simulink model "washing"  (R2024b)
settings: Solver=VariableStepAuto  StartTime=0.0  StopTime=inf  RelTol=1e-3
settings Model: Creator=Dell  LastModifiedBy=Dell

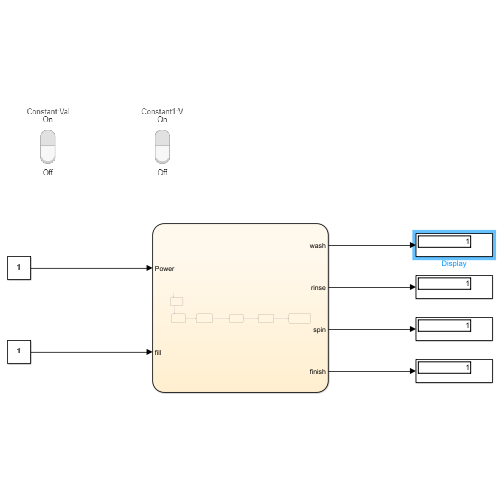
[thumbnail: Simulink's stored preview of the top-level diagram]
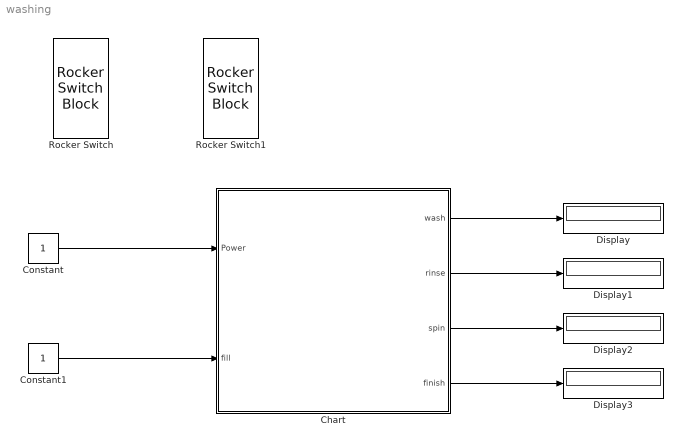
== system washing ==
  Chart : Stateflow chart  TreatAsAtomicUnit=on
  Constant : Constant
  Constant1 : Constant
  Display{,1..3} (4 alike) : Display
  Rocker Switch : RockerSwitchBlock
      settings: Values={{'Off', 'On'}, [0 1]}
  Rocker Switch1 : RockerSwitchBlock
      settings: Values={{'Off', 'On'}, [0 1]}
  wires:
  Constant/1 -> Chart/1(Power)
  Constant1/1 -> Chart/2(fill)
  Chart/2(rinse) -> Display1/1
  Chart/3(spin) -> Display2/1
  Chart/4(finish) -> Display3/1
  Chart/1(wash) -> Display/1

== stateflow chart washing/Chart ==
  state Power_on
  state finish
    entry:finish=1
  state wash
    entry:wash=1
  state fill
  state rinse
    entry:rinse=1
  state spin
    entry:spin=1
  (default) -> Power_on
  Power_on -> fill : [Power==1]
  fill -> wash : [fill==1]
  wash -> rinse : [after(10,sec)]
  rinse -> spin : [after(10,sec)]
  spin -> finish : [after(10,sec)]
  data: wash output; rinse output; spin output; finish output; Power input; fill input
